simulink model "regular_PID"  (R2014a)
settings: Solver=ode15s  StartTime=0.0  StopTime=1500  MaxStep=1000  RelTol=1e-6
PostLoadFcn:
  | cd(fileparts(which(bdroot)))
settings Model: ModifiedByFormat=Mars  ModifiedHistory=Modified by YiXiuKeJi; Taobao is : https://shop197632247.taobao.com  Creator=一休科技  LastModifiedBy=Mars
settings DataIOCC: SignalLoggingSaveFormat=ModelDataLogs  SignalLoggingName=sigsOut
settings OptimizationCC: ExpressionDepthLimit=2147483647  InitFltsAndDblsToZero=on
settings DebuggingCC: SaveWithParameterizedLinksMsg=none  UnderspecifiedInitializationDetection=Classic  SignalResolutionControl=TryResolveAllWithWarning  SolverPrmCheckMsg=none  MultiTaskDSMMsg=warning  MultiTaskCondExecSysMsg=none  FcnCallInpInsideContextMsg=EnableAllAsWarning  FrameProcessingCompatibilityMsg=error  StateNameClashWarn=warning
settings HardwareCC: TargetUnknown=on
settings GRTTargetCC: TargetFcnLib=ansi_tfl_tmw.mat  CombineOutputUpdateFcns=off  GRTInterface=on

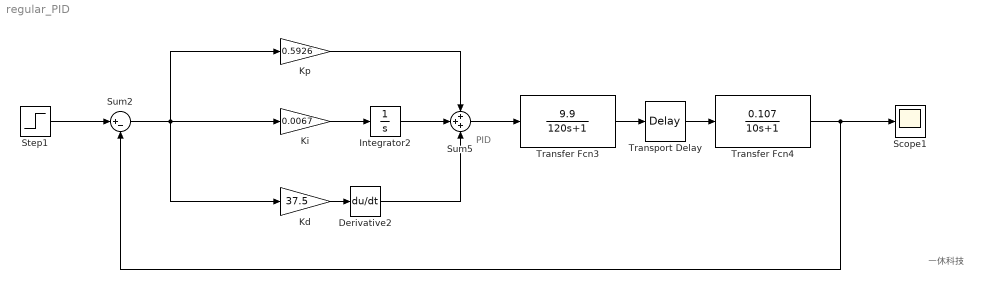
== system regular_PID ==
  note: PID
  note: 一休科技
  Derivative2 : Derivative
  Integrator2 : Integrator
  Kd : Gain  Gain=37.5
  Ki : Gain  Gain=0.0067
  Kp : Gain  Gain=0.5926
  Scope1 : Scope
      settings: TimeRange=auto  MaxDataPoints=5000  SaveToWorkspace=off  YMin=-14.62288  YMax=131.60595  SampleTime=-1
  Step1 : Step  Time=0  After=100  SampleTime=0
  Sum2 : Sum  Inputs=|+-  SaturateOnIntegerOverflow=on
  Sum5 : Sum  Inputs=+++
  Transfer Fcn3 : TransferFcn  Numerator=[9.9 ]  Denominator=[120 1]
  Transfer Fcn4 : TransferFcn  Numerator=[0.107]  Denominator=[10 1]
  Transport Delay : TransportDelay  DelayTime=80
  wires:
  Derivative2/1 -> Sum5/3
  Integrator2/1 -> Sum5/2
  Sum2/1 -> Kd/1, Kp/1, Ki/1
  Sum5/1 -> Transfer Fcn3/1
  Ki/1 -> Integrator2/1
  Transfer Fcn4/1 -> Scope1/1, Sum2/2
  Step1/1 -> Sum2/1
  Transfer Fcn3/1 -> Transport Delay/1
  Transport Delay/1 -> Transfer Fcn4/1
  Kd/1 -> Derivative2/1
  Kp/1 -> Sum5/1
